simulink model "Block_diagram"  (R2023b)
settings: Solver=VariableStepAuto  StartTime=0.0  StopTime=1000  RelTol=1e-3
settings Model: Creator=user  LastModifiedBy=user

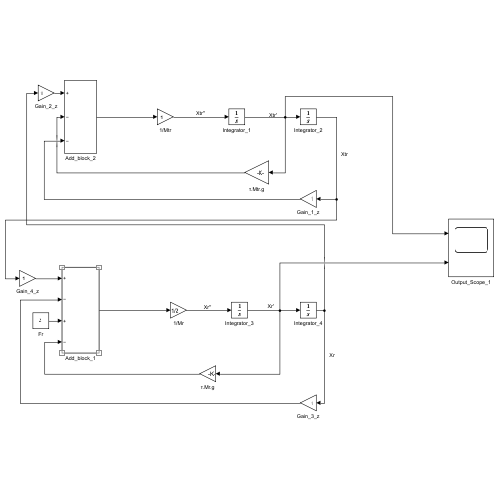
[thumbnail: Simulink's stored preview of the top-level diagram]
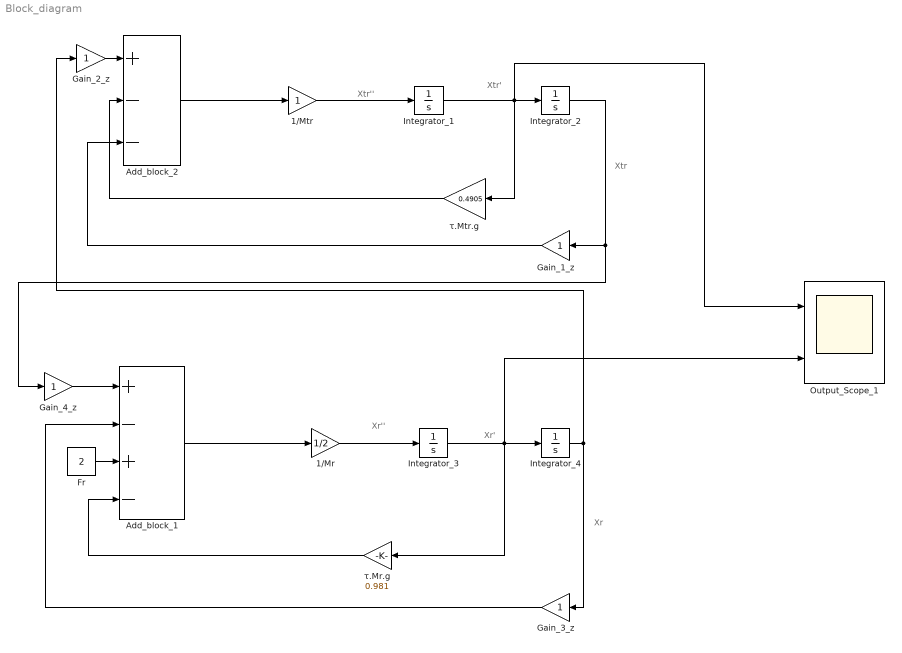
== system Block_diagram ==
  note: Xtr'
  note: Xr'
  note: Xr
  note: Xtr''
  note: Xr''
  note: Xtr
  1/Mr : Gain  Gain=1/2
  1/Mtr : Gain
  Add_block_1 : Sum  Inputs=+-+-
  Add_block_2 : Sum  Inputs=+--
  Fr : Constant  Value=2
  Gain_1_z : Gain
  Gain_2_z : Gain
  Gain_3_z : Gain
  Gain_4_z : Gain
  Integrator_{1..4} (4 alike) : Integrator
  Output_Scope_1 : Scope  NumInputPorts=2
  τ.Mr.g : Gain  Gain=0.981
  τ.Mtr.g : Gain  Gain=0.4905
  wires:
  1/Mtr/1 -> Integrator_1/1
  Integrator_1/1 -> Output_Scope_1/1, τ.Mtr.g/1, Integrator_2/1
  Integrator_2/1 -> Gain_4_z/1, Gain_1_z/1
  Add_block_2/1 -> 1/Mtr/1
  Integrator_3/1 -> Output_Scope_1/2, τ.Mr.g/1, Integrator_4/1
  Gain_3_z/1 -> Add_block_1/2
  1/Mr/1 -> Integrator_3/1
  τ.Mr.g/1 -> Add_block_1/4
  Gain_2_z/1 -> Add_block_2/1
  Fr/1 -> Add_block_1/3
  Add_block_1/1 -> 1/Mr/1
  Integrator_4/1 -> Gain_3_z/1, Gain_2_z/1
  τ.Mtr.g/1 -> Add_block_2/2
  Gain_1_z/1 -> Add_block_2/3
  Gain_4_z/1 -> Add_block_1/1
